simulink model "examen"  (R2022b)
settings: Solver=VariableStepAuto  StartTime=0.0  StopTime=9  RelTol=1e-3
settings Model: Creator=adanaviles  LastModifiedBy=adanaviles

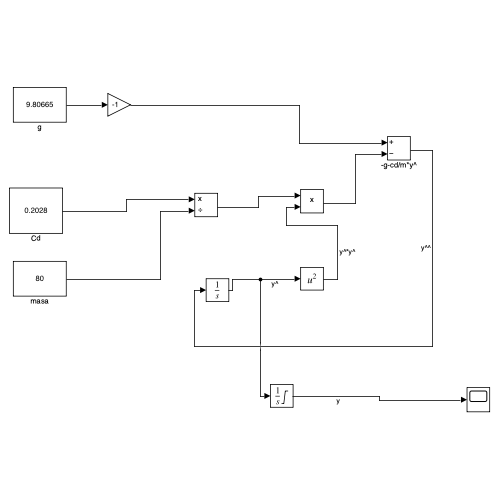
[thumbnail: Simulink's stored preview of the top-level diagram]
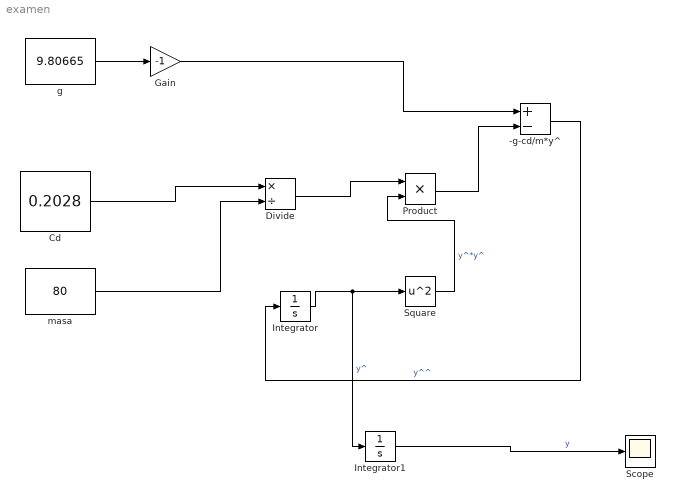
== system examen ==
  -g-cd/m*y^ : Sum  Inputs=+-
  Cd : Constant  Value=0.2028
  Divide : Product  Inputs=*/
  Gain : Gain  Gain=-1
  Integrator : Integrator
  Integrator1 : Integrator  InitialCondition=500  LimitOutput=on  LowerSaturationLimit=0
  Product : Product
  Scope : Scope
  Square : Math  Operator=square
  g : Constant  Value=9.80665
  masa : Constant  Value=80
  wires:
  Cd/1 -> Divide/1
  masa/1 -> Divide/2
  Gain/1 -> -g-cd/m*y^/1
  g/1 -> Gain/1
  Divide/1 -> Product/1
  Product/1 -> -g-cd/m*y^/2
  -g-cd/m*y^/1 -> Integrator/1  "y^^"
  Integrator/1 -> Integrator1/1, Square/1  "y^"
  Square/1 -> Product/2  "y^*y^"
  Integrator1/1 -> Scope/1  "y"
